simulink subsystem "ControlerBA"  (R2023b)
settings: Solver=VariableStepAuto  StartTime=0.0  StopTime=10.0  RelTol=1e-3
settings Model: Creator=Andrés  LastModifiedBy=Andrés

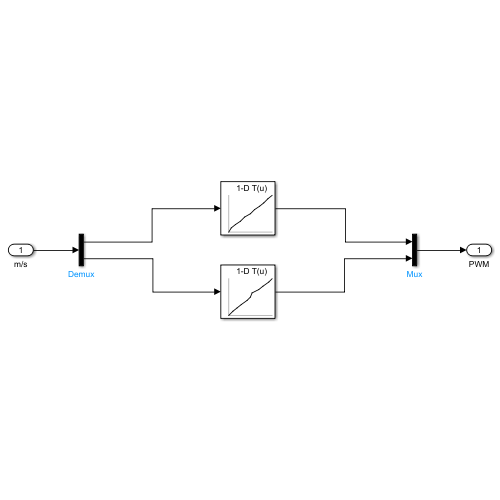
[thumbnail: Simulink's stored preview of the top-level diagram]
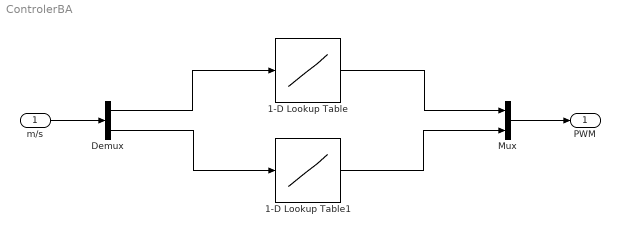
== system ControlerBA ==
  m/s : Inport
  1-D Lookup Table : Lookup_n-D  NumberOfTableDimensions=1  BreakpointsForDimension1=[-0.538387298583984 -0.467544555664063 -0.368366241455078 -0.255023002624512 -0.141679763793945 0 0.0991758108139038 0.226687431335449 0.325862884521484 0.439208984375 0.538375854492188]  Table=[-255 -200 -150 -100 -50 0 50 100 150 200 255]  InternalRulePriority=Speed  RndMeth=Simplest
  1-D Lookup Table1 : Lookup_n-D  NumberOfTableDimensions=1  BreakpointsForDimension1=[-0.538383483886719 -0.425041198730469 -0.325859069824219 -0.2266845703125 -0.0850143432617188 0 0.028335940092802 0.198351860046387 0.311695098876953 0.439205169677734 0.524208068847656]  Table=[-255 -200 -150 -100 -50 0 50 100 150 200 255]  InternalRulePriority=Speed  RndMeth=Simplest
  Demux : Demux  Outputs=2
  Mux : Mux  Inputs=2
  PWM : Outport
  wires:
  m/s/1 -> Demux/1
  Mux/1 -> PWM/1
  Demux/1 -> 1-D Lookup Table/1
  1-D Lookup Table/1 -> Mux/1
  Demux/2 -> 1-D Lookup Table1/1
  1-D Lookup Table1/1 -> Mux/2
